simulink model "Black_Start"  (R2025a)
settings: Solver=FixedStepAuto  StartTime=0.0  StopTime=10.0  FixedStep=Ts  RelTol=1e-3
model mask{referenceFrequency=referenceFrequency, controllerBlackStart=controllerBlackStart, voltageLevel1=voltageLevel1, voltageLevel2=voltageLevel2, voltageLevel3=voltageLevel3, delayLevel1=delayLevel1, delayLevel2=delayLevel2, delayLevel3=delayLevel3}
  mask prompts: referenceFrequency "Reference Frequency"; controllerBlackStart "Black Start Time"; voltageLevel1 "Level1"; voltageLevel2 "Level2"; voltageLevel3 "Level3"; delayLevel1 "Delay1"; delayLevel2 "Delay2"; delayLevel3 "Delay3"
model workspace (MAT data in the model file):
  Ts = 0.001
  controllerBlackStart = 1
  delayLevel1 = 0
  delayLevel2 = 0
  delayLevel3 = 0
  referenceFrequency = 0
  voltageLevel1 = 0
  voltageLevel2 = 0
  voltageLevel3 = 0
undefined symbols (not defined in the file): DiscIntNeverNeededParam
settings Model: ParameterArgumentNames=controllerBlackStart,delayLevel1,delayLevel2,delayLevel3,referenceFrequency,voltageLevel1,voltageLevel2,voltageLevel3  Creator=skota  LastModifiedBy=skota
settings DataIOCC: SaveFormat=StructureWithTime  SaveOutput=off  SignalLogging=off  DSMLogging=off  SaveTime=off  ReturnWorkspaceOutputs=off
settings RTWCC: Toolchain=MinGW64 | CMake/gmake (64-bit Windows)  BuildConfiguration=Release  GPUComputeCapability=3.5

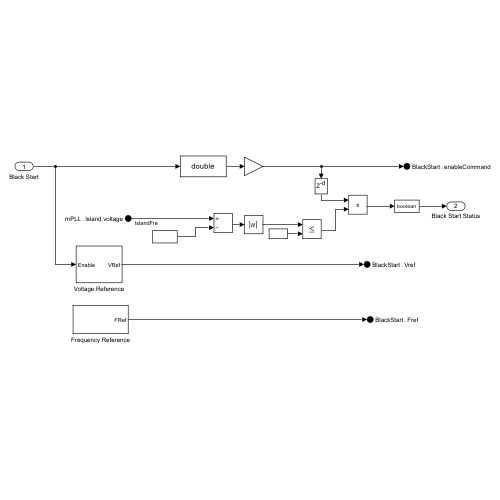
[thumbnail: Simulink's stored preview of the top-level diagram]
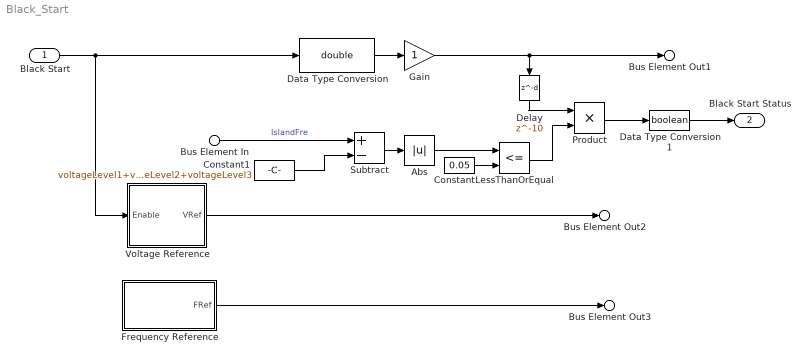
== system Black_Start ==
  Black Start : Inport  OutDataTypeStr=boolean
  Bus Element In : Inport  Port=2  PortName=mPLL  Element=Island.voltage
  Abs : Abs  SaturateOnIntegerOverflow=off
  Constant : Constant  Value=0.05
  Constant1 : Constant  Value=voltageLevel1+voltageLevel2+voltageLevel3
  Data Type Conversion : DataTypeConversion  OutDataTypeStr=double  SaturateOnIntegerOverflow=off  RndMeth=Floor
  Data Type Conversion1 : DataTypeConversion  OutDataTypeStr=boolean  SaturateOnIntegerOverflow=off  RndMeth=Floor
  Delay : Delay  DelayLength=10
  Frequency Reference : Subsystem
  Gain : Gain
  LessThanOrEqual : RelationalOperator  Operator=<=  OutDataTypeStr=boolean  RndMeth=Simplest  InputSameDT=off
  Product : Product
  Subtract : Sum  Inputs=+-
  Voltage Reference : Subsystem
  Bus Element Out2 : Outport  PortName=BlackStart  Element=Vref
  Bus Element Out3 : Outport  PortName=BlackStart  Element=Fref
  Bus Element Out1 : Outport  PortName=BlackStart  Element=enableCommand
  Black Start Status : Outport  Port=2
  wires:
  Gain/1 -> Bus Element Out1/1, Delay/1
  Black Start/1 -> Voltage Reference/1(Enable), Data Type Conversion/1
  Voltage Reference/1(VRef) -> Bus Element Out2/1
  Frequency Reference/1(FRef) -> Bus Element Out3/1
  Data Type Conversion/1 -> Gain/1
  Subtract/1 -> Abs/1
  Product/1 -> Data Type Conversion1/1
  Abs/1 -> LessThanOrEqual/1
  Constant/1 -> LessThanOrEqual/2
  LessThanOrEqual/1 -> Product/2
  Data Type Conversion1/1 -> Black Start Status/1
  Constant1/1 -> Subtract/2
  Bus Element In/1 -> Subtract/1  "IslandFre"
  Delay/1 -> Product/1

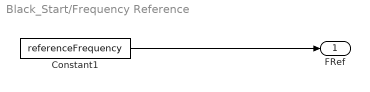
== system Black_Start/Frequency Reference ==
  Constant1 : Constant  Value=referenceFrequency
  FRef : Outport
  wires:
  Constant1/1 -> FRef/1

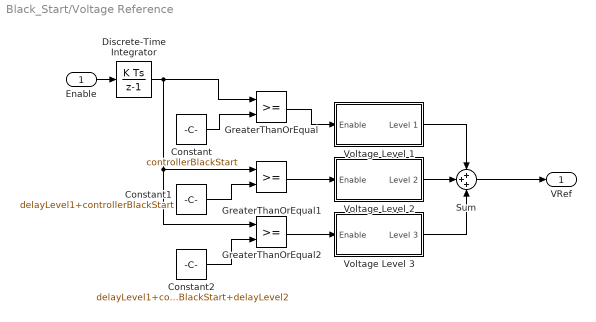
== system Black_Start/Voltage Reference ==
  Enable : Inport
  Constant : Constant  Value=controllerBlackStart
  Constant1 : Constant  Value=delayLevel1+controllerBlackStart
  Constant2 : Constant  Value=delayLevel1+controllerBlackStart+delayLevel2
  Discrete-Time Integrator : DiscreteIntegrator  SampleTime=Ts  OutDataTypeStr=double  ICPrevOutput=DiscIntNeverNeededParam  ICPrevScaledInput=DiscIntNeverNeededParam
  GreaterThanOrEqual : RelationalOperator  OutDataTypeStr=boolean  RndMeth=Simplest  InputSameDT=off
  GreaterThanOrEqual1 : RelationalOperator  OutDataTypeStr=boolean  RndMeth=Simplest  InputSameDT=off
  GreaterThanOrEqual2 : RelationalOperator  OutDataTypeStr=boolean  RndMeth=Simplest  InputSameDT=off
  Sum : Sum  Inputs=+++
  Voltage Level 1 : Subsystem
  Voltage Level 2 : Subsystem
  Voltage Level 3 : Subsystem
  VRef : Outport
  wires:
  Sum/1 -> VRef/1
  Voltage Level 2/1(Level 2) -> Sum/2
  Voltage Level 3/1(Level 3) -> Sum/3
  Voltage Level 1/1(Level 1) -> Sum/1
  GreaterThanOrEqual/1 -> Voltage Level 1/1(Enable)
  GreaterThanOrEqual1/1 -> Voltage Level 2/1(Enable)
  Enable/1 -> Discrete-Time Integrator/1
  Discrete-Time Integrator/1 -> GreaterThanOrEqual2/1, GreaterThanOrEqual1/1, GreaterThanOrEqual/1
  Constant/1 -> GreaterThanOrEqual/2
  Constant1/1 -> GreaterThanOrEqual1/2
  GreaterThanOrEqual2/1 -> Voltage Level 3/1(Enable)
  Constant2/1 -> GreaterThanOrEqual2/2

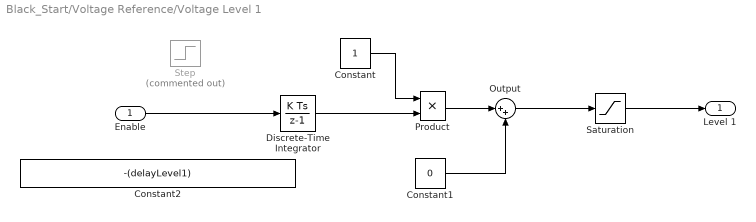
== system Black_Start/Voltage Reference/Voltage Level 1 ==
  Enable : Inport
  Constant : Constant
  Constant1 : Constant  Value=0
  Constant2 : Constant  DisableCoverage=on  Value=-(delayLevel1)  OutDataTypeStr=Inherit: Inherit via back propagation  SampleTime=Ts
  Discrete-Time Integrator : DiscreteIntegrator  SampleTime=Ts  OutDataTypeStr=double  ICPrevOutput=DiscIntNeverNeededParam  ICPrevScaledInput=DiscIntNeverNeededParam
  Output : Sum  Inputs=|++  InputSameDT=on  SaturateOnIntegerOverflow=on  OutDataTypeStr=Inherit: Same as first input
  Product : Product  DisableCoverage=on  InputSameDT=on  SaturateOnIntegerOverflow=on  OutDataTypeStr=Inherit: Same as first input
  Saturation : Saturate  UpperLimit=voltageLevel1  LowerLimit=0
  Step : Step  Commented=on  DisableCoverage=on  Time=controllerBlackStart+delayLevel1  OutDataTypeStr=fixdt('double', 'DataTypeOverride', 'Off')  SampleTime=Ts
  Level 1 : Outport
  wires:
  Discrete-Time Integrator/1 -> Product/2
  Saturation/1 -> Level 1/1
  Product/1 -> Output/1
  Output/1 -> Saturation/1
  Enable/1 -> Discrete-Time Integrator/1
  Constant/1 -> Product/1
  Constant1/1 -> Output/2

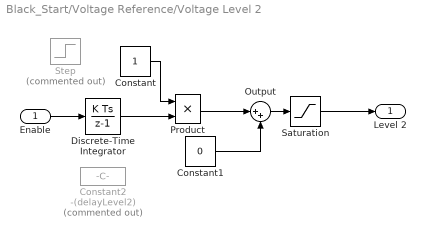
== system Black_Start/Voltage Reference/Voltage Level 2 ==
  Enable : Inport
  Constant : Constant
  Constant1 : Constant  Value=0
  Constant2 : Constant  Commented=on  DisableCoverage=on  Value=-(delayLevel2)  OutDataTypeStr=Inherit: Inherit via back propagation  SampleTime=Ts
  Discrete-Time Integrator : DiscreteIntegrator  SampleTime=Ts  OutDataTypeStr=double  ICPrevOutput=DiscIntNeverNeededParam  ICPrevScaledInput=DiscIntNeverNeededParam
  Output : Sum  Inputs=|++  InputSameDT=on  SaturateOnIntegerOverflow=on  OutDataTypeStr=Inherit: Same as first input
  Product : Product  DisableCoverage=on  InputSameDT=on  SaturateOnIntegerOverflow=on  OutDataTypeStr=Inherit: Same as first input
  Saturation : Saturate  UpperLimit=voltageLevel2  LowerLimit=0
  Step : Step  Commented=on  DisableCoverage=on  Time=delayLevel1+delayLevel2  OutDataTypeStr=fixdt('double', 'DataTypeOverride', 'Off')  SampleTime=Ts
  Level 2 : Outport
  wires:
  Output/1 -> Saturation/1
  Product/1 -> Output/1
  Saturation/1 -> Level 2/1
  Discrete-Time Integrator/1 -> Product/2
  Enable/1 -> Discrete-Time Integrator/1
  Constant/1 -> Product/1
  Constant1/1 -> Output/2

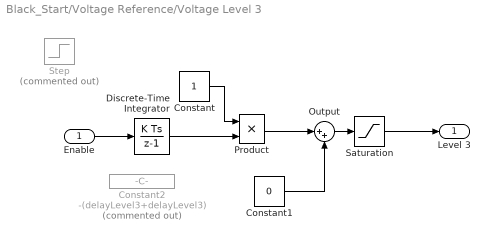
== system Black_Start/Voltage Reference/Voltage Level 3 ==
  Enable : Inport
  Constant : Constant
  Constant1 : Constant  Value=0
  Constant2 : Constant  Commented=on  DisableCoverage=on  Value=-(delayLevel3+delayLevel3)  OutDataTypeStr=Inherit: Inherit via back propagation  SampleTime=Ts
  Discrete-Time Integrator : DiscreteIntegrator  SampleTime=Ts  OutDataTypeStr=double  ICPrevOutput=DiscIntNeverNeededParam  ICPrevScaledInput=DiscIntNeverNeededParam
  Output : Sum  Inputs=|++  InputSameDT=on  SaturateOnIntegerOverflow=on  OutDataTypeStr=Inherit: Same as first input
  Product : Product  DisableCoverage=on  InputSameDT=on  SaturateOnIntegerOverflow=on  OutDataTypeStr=Inherit: Same as first input
  Saturation : Saturate  UpperLimit=voltageLevel3  LowerLimit=0
  Step : Step  Commented=on  DisableCoverage=on  Time=delayLevel1+delayLevel2+delayLevel3  OutDataTypeStr=fixdt('double', 'DataTypeOverride', 'Off')  SampleTime=Ts
  Level 3 : Outport
  wires:
  Discrete-Time Integrator/1 -> Product/2
  Saturation/1 -> Level 3/1
  Product/1 -> Output/1
  Output/1 -> Saturation/1
  Enable/1 -> Discrete-Time Integrator/1
  Constant/1 -> Product/1
  Constant1/1 -> Output/2
